simulink library "HANcoder_STM32_Target2018b"  (R2018b)
settings: Solver=ode45  StartTime=0.0  StopTime=10.0  RelTol=1e-3  EnableMultiTasking=on
libraries: simulink x3
(part 4 of 7)

== system HANcoder_STM32_Target2018b/STM32-E407/UDP ==
  UDP Client Send : Subsystem  Tag=HANcoder_TARGET_STM32_E407  mask(UDP Client Send){ip1=192, ip2=168, ip3=178, ip4=35, port=2000, inputNumber=10, dataType=uint8, byteOrder=on, tsamp=-1}
      mask prompts: ip1 "IP address 1"; ip2 "IP address 2"; ip3 "IP address 3"; ip4 "IP address 4"; inputNumber "Input ports"; dataType "Input datatype"; byteOrder "Byte order: Checked = MSB first, unchecked = LSB first."; tsamp "Sample time"
      mask help:
      | Function
      | ========
      | Sends a data packet to the UDP server with the specified IP address on
      | the specified port.
      |
      | Parameters
      | ==========
      | IP address 1:   First quad of the UDP server's IP address.
      | IP address 2:   Second quad of the UDP server's IP address.
      | IP address 3:   Third quad of the UDP server's IP address.
      | IP address 4:   Fourth quad of the UDP server's IP address.
      | Port:           Port to send the data packet on.
      | Input ports:    The amount of input ports.
      | Input datatype: The datatype of the input ports.
      | Byte order:     Select MSB or LSB first.
      | Sample time:    -1 or divisible by base sample time [seconds].
      |
      | Input
      | =====
      | Port 1..32      UDP packet data.
      mask init:
      | sfcn_udp_client_send_mcb(ip1,ip2,ip3,ip4,port,inputNumber,dataType,byteOrder);
      settings: MoveFcn=drawLogos
      mask Help: web('sfcn_udp_client_send.html');
      mask TypeOptions inputNumber: 1 | 2 | 3 | 4 | 5 | 6 | 7 | 8 | 9 | 10 | 11 | 12 | 13 | 14 | 15 | 16 | 17 | 18 | 19 | 20 | 21 | 22 | 23 | 24 | 25 | 26 | 27 | 28 | 29 | 30 | 31 | 32
      mask TypeOptions dataType: int8 | uint8 | int16 | uint16 | int32 | uint32 | boolean
      mask Display: fprintf('UDP Client Send\n\nport: %d\nip: %d.%d.%d.%d', port, ip1, ip2, ip3, ip4);patch([125 131 131],[8 14 2],[1 0 0]);patch([133 133 139],[14 2 8],[0 0 0.35]);
  UDP Server Init : Subsystem  Tag=HANcoder_TARGET_STM32_E407  mask(UDP Server Init){port=2001}
      mask help:
      | Function
      | ========
      | Initializes the UDP server to listen for and receive data packets on the
      | specified port.
      |
      | Parameters
      | ==========
      | Port:           Port to listen on.
      mask init:
      | sfcn_udp_server_init_mcb(port);
      settings: MoveFcn=drawLogos
      mask Help: web('sfcn_udp_server_init.html');
      mask Display: fprintf('UDP Server Init\n\nport: %d', port);patch([128 134 134],[8 14 2],[1 0 0]);patch([136 136 142],[14 2 8],[0 0 0.35]);
  UDP Server New Data Available : Subsystem  Tag=HANcoder_TARGET_STM32_E407  mask(UDP Server New Data Available){tsamp=-1}
      mask prompts: tsamp "Sample time"
      mask help:
      | Function
      | ========
      | Checks if the UDP server has new data in its internal receive buffer. This
      | new data flag is set each time a data packet is received by the UDP server.
      | It is reset when the application reads data from the receive buffer.
      |
      | Parameters
      | ==========
      | Sample time:    -1 or divisible by base sample time [seconds].
      |
      | Outport
      | ==========
      | 1 if new data is available in the UDP server's receive buffer that hasn't
      | been read yet by the application, 0 otherwise.
      mask init:
      | sfcn_udp_server_new_mcb();
      settings: MoveFcn=drawLogos
      mask Help: web('sfcn_udp_server_new.html');
      mask Display: fprintf('UDP Server New\nData Available');patch([128 134 134],[8 14 2],[1 0 0]);patch([136 136 142],[14 2 8],[0 0 0.35]);
  UDP Server Receive : Subsystem  Tag=HANcoder_TARGET_STM32_E407  mask(UDP Server Receive){outputNumber=10, dataType=uint8, byteOrder=on, startIdx=1, tsamp=-1}
      mask prompts: outputNumber "Output ports"; dataType "Output datatype"; byteOrder "Byte order: Checked = MSB first, unchecked = LSB first."; startIdx "Start index"; tsamp "Sample time"
      mask help:
      | Function
      | ========
      | Reads data from the UDP server's internal receive buffer.
      |
      | Parameters
      | ==========
      | Output ports:    The amount of output ports.
      | Output datatype: The datatype of the output ports.
      | Byte order:      Select MSB or LSB first.
      | Start index:     Start index in the server's buffer to start reading from.
      | Sample time:     -1 or divisible by base sample time [seconds].
      |
      | Output
      | ======
      | Port 1..32       UDP received packet data.
      mask init:
      | sfcn_udp_server_receive_mcb(outputNumber, dataType, byteOrder, startIdx);
      settings: MoveFcn=drawLogos
      mask Help: web('sfcn_udp_server_receive.html');
      mask TypeOptions outputNumber: 1 | 2 | 3 | 4 | 5 | 6 | 7 | 8 | 9 | 10 | 11 | 12 | 13 | 14 | 15 | 16 | 17 | 18 | 19 | 20 | 21 | 22 | 23 | 24 | 25 | 26 | 27 | 28 | 29 | 30 | 31 | 32
      mask TypeOptions dataType: int8 | uint8 | int16 | uint16 | int32 | uint32 | boolean
      mask TypeOptions startIdx: 1 | 2 | 3 | 4 | 5 | 6 | 7 | 8 | 9 | 10 | 11 | 12 | 13 | 14 | 15 | 16 | 17 | 18 | 19 | 20 | 21 | 22 | 23 | 24 | 25 | 26 | 27 | 28 | 29 | 30 | 31 | 32
      mask Display: fprintf('UDP Server Receive');patch([130 136 136],[8 14 2],[1 0 0]);patch([138 138 144],[14 2 8],[0 0 0.35]);
  UDP Server Receive Size : Subsystem  Tag=HANcoder_TARGET_STM32_E407  mask(UDP Server Receive Size){tsamp=-1}
      mask prompts: tsamp "Sample time"
      mask help:
      | Function
      | ========
      | Reads the size in bytes of the last UDP packet that was received by the
      | UDP server and stored in its internal receive buffer.
      |
      | Parameters
      | ==========
      | Sample time:    -1 or divisible by base sample time [seconds].
      |
      | Outport
      | ==========
      | Number of bytes currently stored in the UDP server's receive buffer.
      mask init:
      | sfcn_udp_server_count_mcb();
      settings: MoveFcn=drawLogos
      mask Help: web('sfcn_udp_server_count.html');
      mask Display: fprintf('UDP Server Receive\n Size');patch([128 134 134],[8 14 2],[1 0 0]);patch([136 136 142],[14 2 8],[0 0 0.35]);

== system HANcoder_STM32_Target2018b/STM32-E407/UDS ==
  UDS Get Key : Subsystem  Tag=HANcoder_TARGET_STM32_E407  mask(UDS Get Key){tsamp=-1}
      mask prompts: tsamp "Sample time"
      mask help:
      | Function
      | ==========
      | Reads the 32-bit key value that was received from the UDS tester.
      |
      | Outport
      | =======
      |  - Key value that was received from the UDS tester.
      mask init:
      | sfcn_uds_get_key_mcb();
      settings: MoveFcn=drawLogos
      mask Help: web('sfcn_uds_get_key.html');
      mask Display: fprintf('UDS Get Key');patch([65 71 71],[8 14 2],[1 0 0]);patch([73 73 79],[14 2 8],[0 0 0.35]);
  UDS Get Seed : Subsystem  Tag=HANcoder_TARGET_STM32_E407  mask(UDS Get Seed){tsamp=-1}
      mask prompts: tsamp "Sample time"
      mask help:
      | Function
      | ==========
      | Reads the 32-bit seed value to be used in the seed/key unlock sequence.
      |
      | Outport
      | =======
      |  - Seed value to be used in the seed/key unlock sequence.
      mask init:
      | sfcn_uds_get_seed_mcb();
      settings: MoveFcn=drawLogos
      mask Help: web('sfcn_uds_get_seed.html');
      mask Display: fprintf('UDS Get Seed');patch([65 71 71],[8 14 2],[1 0 0]);patch([73 73 79],[14 2 8],[0 0 0.35]);
  UDS Get Seed Event : Subsystem  Tag=HANcoder_TARGET_STM32_E407  mask(UDS Get Seed Event){}
      mask help:
      | Function
      | ========
      | A 'UDS Get Seed Event' block is needed when the parameter 'UDS seed/key
      | required' is set to TRUE (checked) in the 'UDS Init' block.
      |
      | This block has a function call output that gets triggered during a seed/key
      | sequence, when the UDS module needs a seed. The connected subsystem should
      | contain a 'UDS Set Seed' block to give the seed back to the UDS module.
      |
      | Outport
      | =======
      | Event
      |   Allows connection of a function call subsystem.
      mask init:
      | sfcn_uds_get_seed_event_mcb();
      settings: MoveFcn=drawLogos
      mask Help: web('sfcn_uds_get_seed_event.html');
      mask Display: fprintf('UDS Get Seed Event');patch([95 101 101],[8 14 2],[1 0 0]);patch([103 103 109],[14 2 8],[0 0 0.35]);
  UDS Init : Subsystem  Tag=HANcoder_TARGET_STM32_E407  mask(UDS Init){canChannel=CAN 1, canTxId=hex2dec('7E8'), canRxId=hex2dec('7E0'), tpBlockSize=4, tpSTmin=40, tpRxBuffSize=64, udsTxBuffSize=64, udsUseSeedKey=off}
      mask prompts: canChannel "CAN channel"; canTxId "CAN transmit ID"; canRxId "CAN receive ID"; tpBlockSize "TP blocksize"; tpSTmin "TP STmin"; tpRxBuffSize "TP reception buffer size"; udsTxBuffSize "UDS transmit buffer size"; udsUseSeedKey "UDS seed/key required"
      mask help:
      | Function
      | ==========
      | Initializes the Unified Diagnostic Services (UDS) communication module.
      |
      | Parameters
      | ==========
      | CAN channel: The CAN channel to communicate on
      | CAN transmit ID: CAN identifier for ECU to Tester
      | CAN receive ID: CAN identifier for Tester to ECU
      | TP blocksize: Number of CF's to receive before sending a FC
      | TP STmin: Min separation time (ms) expected between CF's
      | TP reception buffer size: Size of the buffer for TP receptions
      | UDS transmit buffer size: Size of the buffer for UDS/TP transmissions
      | UDS seed/key required: Requires a seed/key unlock sequence
      mask init:
      | sfcn_uds_init_mcb(canChannel, canTxId, canRxId, tpBlockSize, tpSTmin, tpRxBuffSize, udsTxBuffSize, udsUseSeedKey);
      settings: MoveFcn=drawLogos
      mask Help: web('sfcn_uds_init.html');
      mask TypeOptions canChannel: CAN 1 | CAN 2
      mask TypeOptions tpBlockSize: 1 | 2 | 3 | 4 | 5 | 6 | 7 | 8 | 9 | 10 | 11 | 12 | 13 | 14 | 15 | 16 | 17 | 18 | 19 | 20 | 21 | 22 | 23 | 24 | 25 | 26 | 27 | 28 | 29 | 30 | 31 | 32 | 33 | 34 | 35 | 36 | 37 | 38 | 39 | 40 | 41 | 42 | 43 | 44 | 45 | 46 | 47 | 48 | 49 | 50 | 51 | 52 | 53 | 54 | 55 | 56 | 57 | 58 | 59 | 60 | 61 | 62 | 63 | 64 | 65 | 66 | 67 | 68 | 69 | 70 | 71 | 72 | 73 | 74 | 75 | 76 | 77 | 78 | 79 | 80 | 81 | 82 | 83 | 84 | 85 | 86 | 87 | 88 | 89 | 90 | 91 | 92 | 93 | 94 | 95 | 96 | 97 | 98 | 99 | 100 | 101 | 102 | 103 | 104 | 105 | 106 | 107 | 108 | 109 | 110 | 111 | 112 | 113 | 114 | 115 | 116 | 117 | 118 | 119 | 120 | 121 | 122 | 123 | 124 | 125 | 126 | 127 | 128 | 129 | 130 | 131 | 132 | 133 | 134 | 135 | 136 | 137 | 138 | 139 | 140 | 141 | 142 | 143 | 144 | 145 | 146 | 147 | 148 | 149 | 150 | 151 | 152 | 153 | 154 | 155 | 156 | 157 | 158 | 159 | 160 | 161 | 162 | 163 | 164 | 165 | 166 | 167 | 168 | 169 | 170 | 171 | 172 | 173 | 174 | 175 | 176 | 177 | 178 | 179 | 180 | 181 | 182 | 183 | 184 | 185 | 186 | 187 | 188 | 189 | 190 | 191 | 192 | 193 | 194 | 195 | 196 | 197 | 198 | 199 | 200 | 201 | 202 | 203 | 204 | 205 | 206 | 207 | 208 | 209 | 210 | 211 | 212 | 213 | 214 | 215 | 216 | 217 | 218 | 219 | 220 | 221 | 222 | 223 | 224 | 225 | 226 | 227 | 228 | 229 | 230 | 231 | 232 | 233 | 234 | 235 | 236 | 237 | 238 | 239 | 240 | 241 | 242 | 243 | 244 | 245 | 246 | 247 | 248 | 249 | 250 | 251 | 252 | 253 | 254 | 255
      mask TypeOptions tpSTmin: 1 | 2 | 3 | 4 | 5 | 6 | 7 | 8 | 9 | 10 | 11 | 12 | 13 | 14 | 15 | 16 | 17 | 18 | 19 | 20 | 21 | 22 | 23 | 24 | 25 | 26 | 27 | 28 | 29 | 30 | 31 | 32 | 33 | 34 | 35 | 36 | 37 | 38 | 39 | 40 | 41 | 42 | 43 | 44 | 45 | 46 | 47 | 48 | 49 | 50 | 51 | 52 | 53 | 54 | 55 | 56 | 57 | 58 | 59 | 60 | 61 | 62 | 63 | 64 | 65 | 66 | 67 | 68 | 69 | 70 | 71 | 72 | 73 | 74 | 75 | 76 | 77 | 78 | 79 | 80 | 81 | 82 | 83 | 84 | 85 | 86 | 87 | 88 | 89 | 90 | 91 | 92 | 93 | 94 | 95 | 96 | 97 | 98 | 99 | 100 | 101 | 102 | 103 | 104 | 105 | 106 | 107 | 108 | 109 | 110 | 111 | 112 | 113 | 114 | 115 | 116 | 117 | 118 | 119 | 120 | 121 | 122 | 123 | 124 | 125 | 126 | 127 | 128 | 129 | 130 | 131 | 132 | 133 | 134 | 135 | 136 | 137 | 138 | 139 | 140 | 141 | 142 | 143 | 144 | 145 | 146 | 147 | 148 | 149 | 150 | 151 | 152 | 153 | 154 | 155 | 156 | 157 | 158 | 159 | 160 | 161 | 162 | 163 | 164 | 165 | 166 | 167 | 168 | 169 | 170 | 171 | 172 | 173 | 174 | 175 | 176 | 177 | 178 | 179 | 180 | 181 | 182 | 183 | 184 | 185 | 186 | 187 | 188 | 189 | 190 | 191 | 192 | 193 | 194 | 195 | 196 | 197 | 198 | 199 | 200 | 201 | 202 | 203 | 204 | 205 | 206 | 207 | 208 | 209 | 210 | 211 | 212 | 213 | 214 | 215 | 216 | 217 | 218 | 219 | 220 | 221 | 222 | 223 | 224 | 225 | 226 | 227 | 228 | 229 | 230 | 231 | 232 | 233 | 234 | 235 | 236 | 237 | 238 | 239 | 240 | 241 | 242 | 243 | 244 | 245 | 246 | 247 | 248 | 249 | 250 | 251 | 252 | 253 | 254 | 255
      mask Display:
      | fprintf('UDS Init\n(CAN %x)', canChannel);
      | patch([65 71 71],[8 14 2],[1 0 0]);patch([73 73 79],[14 2 8],[0 0 0.35]);
  UDS Set Key Verfied : Subsystem  Tag=HANcoder_TARGET_STM32_E407  mask(UDS Set Key Verified){tsamp=-1}
      mask prompts: tsamp "Sample time"
      mask help:
      | Function
      | ========
      | Informs the UDS module whether or not the key received from the UDS tester
      | is valid.
      |
      | Inport
      | ======
      |  - Set to TRUE in case the key was valid, FALSE otherwise.
      mask init:
      | sfcn_uds_set_key_verified_mcb();
      settings: MoveFcn=drawLogos
      mask Help: web('sfcn_uds_set_key_verified.html');
      mask Display: fprintf('UDS Set Key\nVerified');patch([65 71 71],[8 14 2],[1 0 0]);patch([73 73 79],[14 2 8],[0 0 0.35]);
  UDS Set Seed : Subsystem  Tag=HANcoder_TARGET_STM32_E407  mask(UDS Set Seed){tsamp=-1}
      mask prompts: tsamp "Sample time"
      mask help:
      | Function
      | ==========
      | Sets the 32-bit seed value to be used in the seed/key unlock sequence.
      |
      | Inport
      | ======
      |  - Seed value to be used in the seed/key unlock sequence.
      mask init:
      | sfcn_uds_set_seed_mcb();
      settings: MoveFcn=drawLogos
      mask Help: web('sfcn_uds_set_seed.html');
      mask Display: fprintf('UDS Set Seed');patch([65 71 71],[8 14 2],[1 0 0]);patch([73 73 79],[14 2 8],[0 0 0.35]);
  UDS Verify Key Event : Subsystem  Tag=HANcoder_TARGET_STM32_E407  mask(UDS Verify Key Event){}
      mask help:
      | Function
      | ========
      | A 'UDS Verify Key Event' block is needed when the parameter 'UDS seed/key
      | required' is set to TRUE (checked) in the 'UDS Init' block.
      |
      | This block has a function call output that gets triggered during a seed/key
      | sequence, when the UDS module received a 32-bit key from the tester that
      | needs to be verified. The connected subsystem should contain a 'UDS Set Key
      | Verfied' block to inform the UDS module if the received key was correct.
      |
      | Outport
      | =======
      | Event
      |   Allows connection of a function call subsystem.
      mask init:
      | sfcn_uds_verify_key_event_mcb();
      settings: MoveFcn=drawLogos
      mask Help: web('sfcn_uds_verify_key_event.html');
      mask Display: fprintf('UDS Verify Key Event');patch([95 101 101],[8 14 2],[1 0 0]);patch([103 103 109],[14 2 8],[0 0 0.35]);

== system HANcoder_STM32_Target2018b/STM32-P405/Analog Inputs ==
  Analog Input : Subsystem  Tag=HANcoder_TARGET_STM32_P405  mask(Analog Input){pinID=Port A pin 1, tsamp=-1, filtered=off}
      mask prompts: pinID "Input pin"; tsamp "Sample time"; filtered "Use over sampling and filtering (causes high CPU load)"
      mask help:
      | Function
      | ========
      | Reads the analog/digital conversion results of an analog input pin.
      |
      | Parameters
      | ==========
      | Input pin:
      |   Selects the analog input to read
      |
      | Outport
      | ==========
      | uint16 12-bit conversion results (0-4095).
      mask init:
      | pinIDInfoStr = sfcn_analog_in_mcb(3, pinID,0);
      settings: MoveFcn=drawLogos
      mask Help: web('sfcn_analog_in.html');
      mask TypeOptions pinID: Port A pin 1 | Port B pin 0 | Port B pin 1 | Port C pin 0 | Port C pin 1 | Port C pin 2 | Port C pin 3 | Port C pin 4 | Port C pin 5
      mask Display: fprintf('Analog Input\n%s', pinIDInfoStr);patch([135 141 141],[8 14 2],[1 0 0]);patch([143 143 149],[14 2 8],[0 0 0.35]);

== system HANcoder_STM32_Target2018b/STM32-P405/CAN ==
  CAN : Subsystem
      settings: MoveFcn=drawLogos
      mask Display: fprintf('CAN');patch([85 91 91],[8 14 2],[1 0 0]);patch([93 93 99],[14 2 8],[0 0 0.35]);
  CANopenNode : Subsystem
      settings: MoveFcn=drawLogos
      mask Display: fprintf('CANopenNode');patch([85 91 91],[8 14 2],[1 0 0]);patch([93 93 99],[14 2 8],[0 0 0.35]);

== system HANcoder_STM32_Target2018b/STM32-P405/Digital Inputs ==
  Digital Input : Subsystem  Tag=HANcoder_TARGET_STM32_P405  mask(Digital Input){pinID=Port C pin 10 (5V Tolerant), config=Pulldown, tsamp=-1}
      mask prompts: pinID "Input pin"; config "Configuration"; tsamp "Sample time"
      mask help:
      | Function
      | ========
      | Reads the state of a digital input pin.
      |
      | Parameters
      | ==========
      | Input pin:
      |   Selects the digital input to read
      | Configuration:
      |   Determines if the input is floating or is connected to an internal
      |   pull-up or pull-down resistor.
      |
      | Outport
      | ==========
      | State of the pin. 0 means logical low and 1 logical high
      mask init:
      | pinIDInfoStr = sfcn_digital_in_mcb(3, pinID, config);
      settings: MoveFcn=drawLogos
      mask Help: web('sfcn_digital_in.html');
      mask TypeOptions pinID: Port A pin 1 (5V Tolerant) | Port A pin 8 (5V Tolerant) | Port B pin 0 (5V Tolerant) | Port B pin 1 (5V Tolerant) | Port B pin 2 (5V Tolerant) | Port B pin 5 (5V Tolerant) | Port B pin 8 (5V Tolerant) | Port B pin 9 (5V Tolerant) | Port B pin 10 (5V Tolerant) | Port B pin 11 (5V Tolerant) | Port B pin 12 (5V Tolerant) | Port B pin 13 (5V Tolerant) | Port B pin 14 (5V Tolerant) | Port B pin 15 (5V Tolerant) | Port C pin 0 (5V Tolerant) | Port C pin 1 (5V Tolerant) | Port C pin 2 (5V Tolerant) | Port C pin 3 (5V Tolerant) | Port C pin 4 (5V Tolerant) | Port C pin 5 (5V Tolerant) | Port C pin 6 (5V Tolerant) | Port C pin 7 (5V Tolerant) | Port C pin 8 (5V Tolerant) | Port C pin 9 (5V Tolerant) | Port C pin 10 (5V Tolerant) | Port C pin 11 (5V Tolerant) | Port C pin 12 (5V Tolerant) | Port C pin 13 (5V Tolerant) | Port D pin 2 (5V Tolerant) | Port A pin 0 - BUTTON (5V Tolerant)
      mask TypeOptions config: Floating | Pullup | Pulldown
      mask Display: fprintf('Digital Input\n%s', pinIDInfoStr);patch([135 141 141],[8 14 2],[1 0 0]);patch([143 143 149],[14 2 8],[0 0 0.35]);

== system HANcoder_STM32_Target2018b/STM32-P405/Digital Outputs ==
  Digital Output : Subsystem  Tag=HANcoder_TARGET_STM32_P405  mask(Digital Output){pinID=Port C pin 12 (LED), config=Push pull, tsamp=-1}
      mask prompts: pinID "Output pin"; config "Configuration"; tsamp "Sample time"
      mask help:
      | Function
      | ========
      | Controls the state of a digital output pin.
      |
      | Parameters
      | ==========
      | Output pin:
      |   Selects the digital output to control
      | Configuration:
      |   Open drain (output float when digital high) or push-pull (output connected
      |   to Vcc when digital high).
      |
      | Inport
      | ==========
      | State of the pin. 0 means logical low and 1 logical high
      mask init:
      | pinIDInfoStr = sfcn_digital_out_mcb(3, pinID, config);
      settings: CopyFcn=sfcn_digital_out_chk();  MoveFcn=drawLogos
      mask Help: web('sfcn_digital_out.html');
      mask TypeOptions pinID: Port A pin 1 | Port A pin 8 | Port B pin 0 | Port B pin 1 | Port B pin 2 | Port B pin 5 | Port B pin 8 | Port B pin 9 | Port B pin 10 | Port B pin 11 | Port B pin 12 | Port B pin 13 | Port B pin 14 | Port B pin 15 | Port C pin 0 | Port C pin 1 | Port C pin 2 | Port C pin 3 | Port C pin 4 | Port C pin 5 | Port C pin 6 | Port C pin 7 | Port C pin 8 | Port C pin 9 | Port C pin 10 | Port C pin 11 | Port C pin 12 (LED) | Port C pin 13 | Port D pin 2
      mask Callback pinID: sfcn_digital_out_chk();
      mask TypeOptions config: Open drain | Push pull
      mask Display: fprintf('Digital Output\n%s', pinIDInfoStr);patch([135 141 141],[8 14 2],[1 0 0]);patch([143 143 149],[14 2 8],[0 0 0.35]);

== system HANcoder_STM32_Target2018b/STM32-P405/Error Handling ==
  Clear errors : Subsystem  Tag=HANcoder_TARGET_STM32_P405  mask(Clear errors){eepromString=Active}
      mask prompts: eepromString "Active or Stored error"
      mask help:
      | [Function]
      | Clears the active(RAM) or stored(EEPROM) errors.
      |
      | [Triggerport]
      | Connect the port to a trigger source to execute the block only when necessary.
      mask init:
      | sfcn_controller_error_clearerrors_mcb(eepromString)
      settings: MoveFcn=drawLogos
      mask Help: web('sfcn_controller_error_clearerrors.html');
      mask TypeOptions eepromString: Active | Stored
      mask Display: fprintf('Clear %s Errors', eepromString);patch([80 86 86],[8 14 2],[1 0 0]);patch([88 88 94],[14 2 8],[0 0 0.35]);
  Delete error : Subsystem  Tag=HANcoder_TARGET_STM32_P405  mask(Delete error){useInPorts=off, errorID=hex2dec('8000'), para=10}
      mask prompts: useInPorts "Use inports"; errorID "Error code"; para "Error parameter"
      mask help:
      | [Function]
      | Delete an error defined by error code and parameter
      | from RAM.
      | Error ID and parameter can be specified in the mask or with inports.
      |
      | [Parameters]
      | Error code
      | Error parameter
      |
      | [Inputs]
      | 1 - Error code [uint16]
      | 2 - Error parameter [uint8]
      |
      | [Triggerport]
      | Connect the port to a trigger source to execute the block only when necessary.
      mask init:
      | sfcn_controller_error_deleteerror_mcb(useInPorts, errorID, para)
      settings: MoveFcn=drawLogos
      mask Help: web('sfcn_controller_error_deleteerror.html');
      mask Display: fprintf('Delete error');patch([80 86 86],[8 14 2],[1 0 0]);patch([88 88 94],[14 2 8],[0 0 0.35]);
  Read active error : Subsystem  Tag=HANcoder_TARGET_STM32_P405  mask(Read active error){tsamp=-1}
      mask prompts: tsamp "Sample time"
      mask help:
      | Function
      | ==========
      | Read an active error from RAM.
      |
      | Inport
      | ==========
      | Input is the number of the error in the error list, which can be 1..64. UINT8
      |
      | Outports
      | ==========
      | 1: UINT8 - total amount of errors.
      | 2: UINT16 - error code.
      | 3: UINT8  - error parameter.
      | 4: UINT8  - occurrence count.
      | 5: UINT32 - last occurrence time since startup [milliseconds].
      |
      | Note that the requested error was set and read only if occurrence count > 0.
      mask init:
      | sfcn_controller_error_readerror_mcb(0)
      settings: MoveFcn=drawLogos
      mask Help: web('sfcn_controller_error_readerror.html');
      mask Display: fprintf('Read active error');patch([80 86 86],[8 14 2],[1 0 0]);patch([88 88 94],[14 2 8],[0 0 0.35]);
  Read stored error : Subsystem  Tag=HANcoder_TARGET_STM32_P405  mask(Read stored error){tsamp=-1}
      mask prompts: tsamp "Sample time"
      mask help:
      | Function
      | ==========
      | Read a stored error from EEPROM.
      |
      | Inport
      | ==========
      | Input is the number of the error in the error list, which can be 1..64. UINT8
      |
      | Outports
      | ==========
      | 1: UINT8 - total amount of errors.
      | 2: UINT16 - error code.
      | 3: UINT8  - error parameter.
      | 4: UINT8  - occurrence count.
      | 5: UINT32 - last occurrence time since startup [milliseconds].
      |
      | Note that the requested error was set and read only if occurrence count > 0.
      mask init:
      | sfcn_controller_error_readerror_mcb(1)
      settings: MoveFcn=drawLogos
      mask Help: web('sfcn_controller_error_readerror.html');
      mask Display: fprintf('Read stored error');patch([80 86 86],[8 14 2],[1 0 0]);patch([88 88 94],[14 2 8],[0 0 0.35]);
  Search active error : Subsystem  Tag=HANcoder_TARGET_STM32_P405  mask(Search active error){tsamp=-1}
      mask prompts: tsamp "Sample time"
      mask help:
      | Function
      | ==========
      | Searches for the erorr with the specified error Code and Param in RAM.
      |
      | Inport
      | ==========
      | 1: UINT16 - Error Code
      | 2: UINT8   - Error Parameter
      |
      | Outports
      | ==========
      | 1: UINT8   - occurrence count.
      | 2: UINT32 - last occurrence time since startup [milliseconds]
      |
      | Note that when occurrence count equals zero, the error is not found.
      mask init:
      | sfcn_controller_error_searcherror_mcb(0)
      settings: MoveFcn=drawLogos
      mask Help: web('sfcn_controller_error_searcherror.html');
      mask Display: fprintf('Search active error');patch([80 86 86],[8 14 2],[1 0 0]);patch([88 88 94],[14 2 8],[0 0 0.35]);
  Search stored error : Subsystem  Tag=HANcoder_TARGET_STM32_P405  mask(Search stored error){tsamp=-1}
      mask prompts: tsamp "Sample time"
      mask help:
      | Function
      | ==========
      | Searches for the erorr with the specified error Code and Param in EEPROM.
      |
      | Inport
      | ==========
      | 1: UINT16 - Error Code
      | 2: UINT8   - Error Parameter
      |
      | Outports
      | ==========
      | 1: UINT8   - occurrence count.
      | 2: UINT32 - last occurrence time since startup [milliseconds]
      |
      | Note that when occurrence count equals zero, the error is not found.
      mask init:
      | sfcn_controller_error_searcherror_mcb(1)
      settings: MoveFcn=drawLogos
      mask Help: web('sfcn_controller_error_searcherror.html');
      mask Display: fprintf('Search stored error');patch([80 86 86],[8 14 2],[1 0 0]);patch([88 88 94],[14 2 8],[0 0 0.35]);
  "Store error " : Subsystem  Tag=HANcoder_TARGET_STM32_P405  mask(Store error){useInPorts=off, errorCode=hex2dec('8000'), parameter=10}
      mask prompts: useInPorts "Use inports"; errorCode "Error code"
      mask help:
      | [Function]
      | Store an error to RAM (and EEPROM if new) of the controller.
      | Error ID and parameter can be specified in the mask or with inports.
      |
      | [Parameters]
      | Error code
      | Error parameter
      |
      | [Inputs]
      | 1 - Error code [uint16]
      | 2 - Error parameter [uint8]
      |
      | [Triggerport]
      | Connect the port to a trigger source to execute the block only when necessary.
      mask init:
      | sfcn_controller_error_storeerror_in_mcb(useInPorts, errorCode, parameter, 1)
      settings: MoveFcn=drawLogos
      mask Help: web('sfcn_controller_error_storeerror.html');
      mask Display: fprintf('Store error');patch([80 86 86],[8 14 2],[1 0 0]);patch([88 88 94],[14 2 8],[0 0 0.35]);
  Total Errors : Subsystem  Tag=HANcoder_TARGET_STM32_P405  mask(Total active or stored errors){eepromString=Active, tsamp=-1}
      mask prompts: eepromString "Active or Stored error"; tsamp "Sample time"
      mask help:
      | [Function]
      | Returns the total amount of active or stored errors
      |
      | [Parameters]
      | Active or Stored error [-]
      | sampleTime: [s]
      |
      | [Outputs]
      | Port 1 :Total number of errors [uint8]
      | Port 2 :Highest occuring severity [uint8]
      mask init:
      | sfcn_controller_error_totalerrors_mcb(eepromString, tsamp);
      settings: MoveFcn=drawLogos
      mask Help: web('sfcn_controller_error_totalerrors.html');
      mask TypeOptions eepromString: Active | Stored
      mask Display: fprintf('Total %s Errors', eepromString);patch([80 86 86],[8 14 2],[1 0 0]);patch([88 88 94],[14 2 8],[0 0 0.35]);

== system HANcoder_STM32_Target2018b/STM32-P405/File Logger ==
  File Logger Close : Subsystem  Tag=HANcoder_TARGET_STM32_P405  mask(File Logger Close){}
      mask help:
      | Function
      | ========
      | With the File Logger module active, the data values of the configured signals
      | are sampled at a fixed time interval and written to the log-file on the SD-card.
      |
      | The log-file needs to be explicitly closed at the end of a logging session for the
      | log-file to actually appear on the SD-card.
      |
      | Ideally, this block is called during software shutdown for example when the ignition
      | signal goes low in automotive applications. An external trigger can also be used such
      | as a button press event or CAN message reception.
      |
      | Triggerport
      | ===========
      | Connect the port to a trigger source to execute the block only when necessary.
      mask init:
      | sfcn_filelogger_close_mcb();
      settings: MoveFcn=drawLogos
      mask Help: web('sfcn_filelogger_close.html')
      mask Display: fprintf('File Logger Close');patch([80 86 86],[8 14 2],[1 0 0]);patch([88 88 94],[14 2 8],[0 0 0.35]);
  File Logger Init : Subsystem  Tag=HANcoder_TARGET_STM32_P405  mask(File Logger Init){filename=file.txt, interval=100, fileLoggerMaxFileLength=30, autostart=off, dotseparator=off}
      mask prompts: interval "Logging interval (ms)"; fileLoggerMaxFileLength "Maximum log file size (in KB)"; autostart "Automatically start logging"; dotseparator "Use dot-character as decimal separator (comma otherwise)"
      mask help:
      | Function
      | ==========
      | Initializes the File Logger module to log on the SDcard.
      |
      | Parameters per channel
      | ======================
      | - Filename for the log-file (a number will be added at the end of
      |   the filename for each new logfile)
      | - Logging interval in milliseconds
      | - Maximum size of the log file, a new log file will be started each time
      |   the file size is reached.
      | - Select if logging should automatically start after reset. If not then
      |   logging can be started using the trigger input.
      | - Select if a comma or dot should be used a the decimal point in numbers
      |
      | Note: Use the 'File Logger Close' block to save the data to the SDcard
      mask init:
      | sfcn_filelogger_init_mcb(filename, interval, dotseparator, autostart, fileLoggerMaxFileLength);
      settings: MoveFcn=drawLogos
      mask Help: web('sfcn_filelogger_init.html')
      mask Display: fprintf('File Logger Init');patch([95 101 101],[8 14 2],[1 0 0]);patch([103 103 109],[14 2 8],[0 0 0.35]);
  File Logger Signal : Subsystem  Tag=HANcoder_TARGET_STM32_P405  mask(File Logger Signal){signalName=enter name, dataType=uint8, defineColumns=off, columnNr=1}
      mask prompts: signalName "Signal Name"; dataType "Signal Data Type"; defineColumns "Define ALL column numbers manually"; columnNr "Column number starting at 1:"
      mask help:
      | Function
      | ==========
      | Configures the signal to be logged by the File Logger module.
      |
      | Parameters per channel
      | ======================
      | - Select the name for in the first line of the log file.
      | - Select the data type of the signal.
      | - Check if you want to give a column number to the signal or let Simulink
      |   automatically do it.
      | - Indicate the column in the logfile where this signal's data should be
      |   present (Note: you have to do all of your logged signals)
      settings: MoveFcn=drawLogos
      mask Help: web('sfcn_filelogger_signal.html')
      mask TypeOptions dataType: double | single | int8 | uint8 | int16 | uint16 | int32 | uint32
      mask Callback defineColumns:
      | if strcmp(get_param(gcb, 'defineColumns'),'on')
      | 	set_param(gcb, 'MaskVisibilities',{'on' 'on' 'on' 'on'});
      | else
      |     set_param(gcb, 'MaskVisibilities',{'on' 'on' 'on' 'off'});
      | end
      mask Display:
      | switch dataType
      |     case 1
      |         dataTypeStr = 'double';
      |     case 2
      |         dataTypeStr = 'single';
      |     case 3
      |         dataTypeStr = 'int8';
      |     case 4
      |         dataTypeStr = 'uint8';
      |     case 5
      |         dataTypeStr = 'int16';
      |     case 6
      |         dataTypeStr = 'uint16';
      |     case 7
      |         dataTypeStr = 'int32';
      |     case 8
      |         dataTypeStr = 'uint32';
      |     case 9
      |         dataTypeStr = 'boolean';
      | end
      | fprintf('File Logger Signal\n%s (%s)', signalName, dataTypeStr);patch([110 116 116],[8 14 2],[1 0 0]);patch([118 118 124],[14 2 8],[0 0 0.35]);

== system HANcoder_STM32_Target2018b/STM32-P405/Memory ==
  EEPROM : Subsystem
      settings: MoveFcn=drawLogos
      mask Display: fprintf('EEPROM');patch([85 91 91],[8 14 2],[1 0 0]);patch([93 93 99],[14 2 8],[0 0 0.35]);

== system HANcoder_STM32_Target2018b/STM32-P405/PWM Outputs ==
  PWM Duty Cycle : Subsystem  Tag=HANcoder_TARGET_STM32_P405  mask(Pulse Width Modulation Set Duty Cycle){pinID=Port A pin 9, tsamp=-1}
      mask prompts: pinID "Output pin"; tsamp "Sample time"
      mask help:
      | Function
      | ========
      | A 'PWM Duty Cycle' block allows the duty cycle of the generated PWM signal to
      | changed.
      | Note that this only works properly if a 'PWM Init' block is also present
      | for initializing the related PWM module.
      |
      | Parameters
      | ==========
      | PWM pin:
      |   Selects the PWM pin for which the duty cycle should be updated.
      |
      | Inport
      | ==========
      | uint16 10-bit unsigned value (0..1023) to represent the duty cycle (0..100%) for
      | each enabled channel.
      mask init:
      | pinIDInfoStr = sfcn_pwmout_setduty_mcb(3, pinID);
      settings: MoveFcn=drawLogos
      mask Help: web('sfcn_pwmout_setduty.html');
      mask TypeOptions pinID: Port A pin 8 | Port A pin 9 | Port A pin 10 | Port A pin 1 | Port C pin 6 | Port C pin 7 | Port C pin 8 | Port C pin 9 | Port B pin 6 | Port B pin 7 | Port B pin 8 | Port B pin 9
      mask Display: fprintf('PWM Set Duty Cycle\n%s', pinIDInfoStr);patch([135 141 141],[8 14 2],[1 0 0]);patch([143 143 149],[14 2 8],[0 0 0.35]);
  PWM Init : Subsystem  Tag=HANcoder_TARGET_STM32_P405  mask(Pulse Width Modulation Initialization){moduleID=TIM1: PA8 & PA9 & PA10 & n/a + N-channels PB13 & PB0 & PB1), frequency=10253, alignment=Edge aligned, enableIRQoutput=off, ch1On=off, ch1Pol=Active high, ch1Inv=off, ch2On=off, ch2Pol=Active high, ch2Inv=off, ch3On=off, ch3Pol=Active high, ch3Inv=off, ch4On=off, ch4Pol=Active high, ch4Inv=off}
      mask prompts: moduleID "PWM module"; frequency "Signal frequency [Hz]"; alignment "Signal alignment"; enableIRQoutput "Enable IRQ output"; ch1On "Generate PWM signal on channel 1"; ch1Pol "Select signal polarity"; ch1Inv "Enable inverted signal on additional output pin"; ch2On "Generate PWM signal on channel 2"; ch2Pol "Select signal polarity"; ch2Inv "Enable inverted signal on additional output pin"; ch3On "Generate PWM signal on channel 3"; ch3Pol "Select signal polarity"; ch3Inv "Enable inverted signal on additional output pin"; ch4On "Generate PWM signal on channel 4"; ch4Pol "Select signal polarity"; ch4Inv "Enable inverted signal on additional output pin"
      mask help:
      | Function
      | ========
      | A 'PWM Init' block configures one of the STM32 timer modules for PWM
      | functionality, allowing a PWM signal to be generated on up to 4 timer
      | channels and their associated output pins.
      |
      | Parameters
      | ==========
      | General - PWM module:
      |   Select the PWM module to use. The name in the combo box contains
      |   information about which pins on the target belong to this timer module.
      |   Also the first pin corresponds with the first channel and so on:
      |   TIMx: Ch1 & Ch2 & Ch3...
      |
      | General - Signal frequency:
      |   Determines the signal frequency in Hz. If you click 'Apply' after entering
      |   the desired frequency it will automatically be adjusted to the closest
      |   supported value.
      |
      | General - Signal Aligment:
      |   Determines the aligment of the signal. It can either be edge aligned or
      |   center aligned.
      |
      | General - Enable IRQ output
      |   Controls whether or not the IRQ output is available.
      |
      | Channel x - Generate PWM signal on channel x:
      |   Enable to configure the channel for PWM functionality so that the PWM signal
      |   is outputted on the channel's associated microcontroller pin.
      |
      | Channel x - Signal polarity:
      |   Selects the polarity of the signal.
      |
      | Channel x - Enable inverted signal on additional output pin:
      |   When enabled, a second PWM signal will be generated on an additional
      |   microcontroller pin where the signal is an exact inversion of the first signal.
      mask init:
      | moduleIDInfoStr = sfcn_pwmout_init_mcb(3, moduleID, frequency, alignment, enableIRQoutput, ch1On, ch2On, ch3On, ch4On, ch1Pol, ch2Pol, ch3Pol, ch4Pol, ch1Inv, ch2Inv, ch3Inv, ch4Inv);
      settings: CopyFcn=sfcn_pwmout_init_chk();  MoveFcn=drawLogos
      mask Help: web('sfcn_pwmout_init.html');
      mask TypeOptions moduleID: TIM1: PA8 & PA9 & PA10 & n/a + N-channels PB13 & PB0 & PB1) | TIM2:n/a & PA1 & n/a & n/a | TIM3: PC6 & PC7 & PC8 & PC9 | TIM4: PB6 & PB7 & PC8 & PB9
      mask Callback moduleID: sfcn_pwmout_init_chk();
      mask TypeOptions alignment: Edge aligned | Center aligned
      mask TypeOptions ch1Pol: Active high | Active low
      mask TypeOptions ch2Pol: Active high | Active low
      mask TypeOptions ch3Pol: Active high | Active low
      mask TypeOptions ch4Pol: Active high | Active low
      mask Display: fprintf('PWM Init\n%s', moduleIDInfoStr);patch([185 191 191],[8 14 2],[1 0 0]);patch([193 193 199],[14 2 8],[0 0 0.35]);

== system HANcoder_STM32_Target2018b/STM32-P405/SPI ==
  SPI master init : Subsystem  Tag=HANcoder_TARGET_STM32_P405  mask(SPI master init){channel=SPI1: UEXT 9 & 7 & 8 (PA5 & PA6 & PA7), speed=5250 kHz, polarity=Idle low, phase=Sample bit on 1st clock edge}
      mask prompts: speed "Communication speed"
      mask help:
      | Function
      | ==========
      | Initialized a SPI master channel.
      |
      | Parameters per channel
      | ======================
      | - Select channel
      | - Select communication speed
      | - Select clock signal polarity
      | - Select clock phase to sample a bit
      mask init:
      | spiChannelInfoStr = sfcn_spi_master_init_mcb(3, channel, speed, polarity, phase);
      settings: CopyFcn=sfcn_spi_master_init_chk();  MoveFcn=drawLogos
      mask Help: web('sfcn_spi_master_init.html')
      mask TypeOptions channel: SPI1: UEXT 9 & 7 & 8 (PA5 & PA6 & PA7) | SPI2: PB13 & PB14 & PB15
      mask Callback channel: sfcn_spi_master_init_chk();
      mask TypeOptions speed: 21000 kHz | 10500 kHz | 5250 kHz | 2625 kHz | 1312.5 kHz | 656.25 kHz | 328.125 kHz | 164.0625 kHz
      mask TypeOptions polarity: Idle low | Idle high
      mask TypeOptions phase: Sample bit on 1st clock edge | Sample bit on 2nd clock edge
      mask Display: fprintf('SPI master init\n%s', spiChannelInfoStr);patch([211 217 217],[8 14 2],[1 0 0]);patch([219 219 225],[14 2 8],[0 0 0.35]);
  SPI master transfer : Subsystem  Tag=HANcoder_TARGET_STM32_P405  Priority=1  mask(SPI master transfer){channel=SPI1: UEXT 9 & 7 & 8 (PA5 & PA6 & PA7), useSS=off, SSpin=Port A pin 1, SSenable=on, SSdisable=on, delayCycles=0, userPriority=1, tsamp=-1}
      mask prompts: useSS "Use slave select output"; SSpin "Slave select output pin"; SSenable "Enable slave select before transfer"; SSdisable "Disable slave select after transfer"; delayCycles "Delay cycles between slave select enable and transfer"; userPriority "Priority (use to set order of byte transfer, lowest number is executed first)"; tsamp "Sample time"
      mask help:
      | Function
      | ==========
      | Performs a byte transfer via SPI.
      |
      | Parameters per channel
      | ======================
      | - Select channel
      | - Select if a Slave Select output should be controlled
      |   * Select the Slave Select digital output pin
      |   * Select if the Slave Select should be made logic low before the transfer
      |   * Select if the Slave Select should be made logic high after the transfer
      |   * Enter the number of CPU cycles to delay between Slave Select enable and the transfer
      |
      | Inputs
      | ======
      | The byte value to send to the slave.
      |
      | Outputs
      | =======
      | The byte value received from the slave.
      mask init:
      | spiChannelInfoStr = sfcn_spi_master_transfer_mcb(3, channel, useSS, SSpin, SSenable, SSdisable, delayCycles);
      settings: MoveFcn=drawLogos
      mask Help: web('sfcn_spi_master_transfer.html')
      mask TypeOptions channel: SPI1: UEXT 9 & 7 & 8 (PA5 & PA6 & PA7) | SPI2: PB13 & PB14 & PB15
      mask Callback useSS:
      | % Get the mask parameter
      | useSS = get_param(gcb,'useSS');
      | 
      | if strcmp(useSS,'on')
      |     set_param(gcb,'MaskVisibilities',{'on','on','on','on','on','on','on','on'});
      | else
      |     set_param(gcb,'MaskVisibilities',{'on','on','off','off','off','off','on','on'});
      | end
      mask TypeOptions SSpin: Port A pin 1 | Port A pin 8 | Port B pin 0 | Port B pin 1 | Port B pin 2 | Port B pin 5 | Port B pin 8 | Port B pin 9 | Port B pin 10 | Port B pin 11 | Port B pin 12 | Port B pin 13 | Port B pin 14 | Port B pin 15 | Port C pin 0 | Port C pin 1 | Port C pin 2 | Port C pin 3 | Port C pin 4 | Port C pin 5 | Port C pin 6 | Port C pin 7 | Port C pin 8 | Port C pin 9 | Port C pin 10 | Port C pin 11 | Port C pin 12 (LED) | Port C pin 13 | Port D pin 2
      mask Callback userPriority:
      | userPriority = get_param(gcb, 'userPriority');
      | set_param(gcb,'Priority',userPriority);
      mask Display: fprintf('SPI master transfer\n%s', spiChannelInfoStr);patch([210 216 216],[8 14 2],[1 0 0]);patch([218 218 224],[14 2 8],[0 0 0.35]);

== system HANcoder_STM32_Target2018b/STM32-P405/System Config ==
  Base Sample Time config : Subsystem  Tag=HANcoder_TARGET_STM32_P405  Description=HANcoder Target STM32-P405 blockset version 1.1  mask(Base Sample Time config){baseSampleTime=10, extraStack=100}
      mask prompts: baseSampleTime "Define the base sample time [ms]"; extraStack "Additional task stack (bytes):"
      mask help:
      | Function
      | ==========
      | Sets the Base Sample Time in the model, and automatically sets the sample
      | time in the solver step time menu when the model is simulated or build.
      |
      | Parameters
      | ==========
      | Base Sample Time [milliseconds]
      | Default:    10[ms]
      | Min:        0.1[ms]
      |
      | Note: This is the only block where sample time is set in miliseconds,
      | all other blocks work with sample time in seconds
      |
      | It is possible to reserve extra stack space for the OS task that executes
      | the model on the embedded target (AppCtrlTask).
      mask init:
      | sfcn_base_sample_time_mcb(baseSampleTime*1000, extraStack, 3);
      | HANcoderStruct = get_param(gcb,'UserData');
      | BlocksetVersion = HANcoderStruct.BlocksetVersion;
      settings: MoveFcn=drawLogos
      mask Help: web('sfcn_base_sample_time.html')
      mask Display: fprintf('Blockset version %s\nBase Sample Time:\n %gms',BlocksetVersion,baseSampleTime);patch([91 97 97],[8 14 2],[1 0 0]);patch([99 99 105],[14 2 8],[0 0 0.35]);
  Build settings : Subsystem  Tag=HANcoder_TARGET_STM32_P405  mask(Build Settings){AutoASAP2add=on, AutoFlash=USB}
      mask prompts: AutoASAP2add "Add signals and parameters automatically"; AutoFlash "Automatic flash after build"
      mask help:
      | Function
      | ==========
      | Auto Add:
      | Here you can turn the automatic adding of Signals and Parameters on or off. If the option is on all the parameters and signals which are not defined in the workspace will be added. You will be prompted for the value.
      |
      | Auto Flash:
      | This option will automatically start MicroBoot with the selected interface.
      settings: MoveFcn=drawLogos
      mask Help: web('build_settings.html')
      mask TypeOptions AutoASAP2add: on | off
      mask TypeOptions AutoFlash: off | USB | CAN
      mask DialogControl ParameterTabVar0 Prompt: Auto Add
      mask DialogControl Control3 Prompt: With this option the undefined parameters and signals will automatically be added to the workspace for use with HANtune. You will be prompted for the parameter values.
      mask DialogControl ParameterTabVar01 Prompt: Auto Flash
      mask DialogControl Control2 Prompt: With this option you can choose to automatically start MicroBoot after the build is complete. MicroBoot will start flashing using the selected interface.
      mask Display: fprintf('Build settings\nAuto Add: %s\nAuto Flash: %s',AutoASAP2add, AutoFlash);patch([114 120 120],[8 14 2],[1 0 0]);patch([122 122 128],[14 2 8],[0 0 0.35]);
  CAN config : Subsystem  Tag=HANcoder_TARGET_STM32_P405  mask(CAN config){txBufSize=64, evBufSize=8, canBus1=on, baudRate1=500, rxMask1=hex2dec('00000000'), rxCode1=hex2dec('00000000'), rxMode1=Receive only 11-bit message identifiers, canBus2=off, baudRate2=500, rxMask2=hex2dec('00000000'), rxCode2=hex2dec('00000000'), rxMode2=Receive only 11-bit message identifiers}
      mask prompts: txBufSize "Transmit buffer size CAN bus (max 512)"; evBufSize "Event buffer size CAN bus (max 16)"; canBus1 "Use CAN bus 1"; baudRate1 "Baudrate CAN bus 1 (kbit/s)"; rxMask1 "Reception filter Mask CAN bus 1"; rxCode1 "Reception filter Code CAN bus 1"; rxMode1 "Reception filter Mode CAN bus 1"; canBus2 "Use CAN bus 2"; baudRate2 "Baudrate CAN bus 2 (kbit/s)"; rxMask2 "Reception filter Mask CAN bus 2"; rxCode2 "Reception filter Code CAN bus 2"; rxMode2 "Reception filter Mode CAN bus 2"
      mask help:
      | Function
      | ==========
      | Configures the settings for the STM32's CAN busses.
      |
      | Parameters per channel
      | ======================
      | - Activate channel
      | - Select baud rate (default 500[kbit/s])
      | - Select reception acceptance filter Code
      | - Select reception acceptance filter Mask
      | - Select reception acceptance filter Mode
      mask init:
      | sfcn_can_config_mcb(txBufSize, evBufSize, canBus1, baudRate1, rxMask1, rxCode1, rxMode1, canBus2, baudRate2, rxMask2, rxCode2, rxMode2);
      settings: MoveFcn=drawLogos
      mask Help: web('sfcn_can_config.html')
      mask TypeOptions baudRate1: 125 | 250 | 500 | 1000
      mask TypeOptions rxMode1: Receive only 11-bit message identifiers | Receive only 29-bit message identifiers | Received both 11- and 29-bit message identifiers
      mask TypeOptions baudRate2: 125 | 250 | 500 | 1000
      mask TypeOptions rxMode2: Receive only 11-bit message identifiers | Receive only 29-bit message identifiers | Received both 11- and 29-bit message identifiers
      mask DialogControl ParameterTabVar0 Prompt: Generic
      mask DialogControl ParameterTabVar01 Prompt: CAN 1
      mask DialogControl ParameterTabVar012 Prompt: CAN 2
      mask Display: fprintf('CAN1 : %x\nCAN2 : %x',canBus1, canBus2);patch([58 64 64],[8 14 2],[1 0 0]);patch([66 66 72],[14 2 8],[0 0 0.35]);
  Custom ID config : Subsystem  Tag=HANcoder_TARGET_STM32_P405  mask(Custom ID config){softID=softwareID, softNUM=1}
      mask prompts: softID "Software ID Name"; softNUM "Software Version Number"
      mask help:
      | Function:
      | =========
      | This block can be used to override the generated software ID as the current software version which is used for identification purposes.
      | It can also be used to add a version number behind the software ID.
      |
      | Details:
      | ========
      | If only a software version number is filled in, a software ID will be generated and the version number will be placed behind it.
      | Atleast one pf the fields has to be filled in.
      |
      | Parameters:
      | ===========
      | Software ID name:
      | Fill in the desired custom ID. Must fit in a UINT8
      | Software Version Number:
      | Fill in the desired version number. Must fit in a UINT8
      mask init:
      | sfcn_custom_version_config_mcb(softID, softNUM)
      settings: MoveFcn=drawLogos
      mask Help: web('sfcn_custom_ID_config.html')
      mask Display: fprintf('Custom software ID:\n "%s"\n Software version:\n "%s"', char(softID), char(softNUM));patch([112 118 118],[8 14 2],[1 0 0]);patch([120 120 126],[14 2 8],[0 0 0.35]);
  XCP on CAN config : Subsystem  Tag=HANcoder_TARGET_STM32_P405  mask(XCP on CAN config){canBus=CAN 1, croID=hex2dec('665'), dtoID=hex2dec('666')}
      mask prompts: canBus "CAN channel"; croID "CRO identifier"; dtoID "DTO identifier"
      mask help:
      | Function
      | ==========
      | Implements XCP communication into your application using the CAN network.
      |
      | Parameter
      | ==========
      | Specify the CAN channel to be used for XCP.
      | Specify the CAN CRO message identifier for XCP (master->slave).
      | Specify the CAN DTO message identifier for XCP (slave->master).
      |
      | Notes
      | ==========
      | Baudrates can be modified in the CAN config block.
      mask init:
      | sfcn_can_xcp_config_mcb(canBus, croID, dtoID)
      settings: MoveFcn=drawLogos
      mask Help: web('sfcn_can_xcp_config.html')
      mask TypeOptions canBus: CAN 1 | CAN 2
      mask Display: fprintf('XCP over CAN: %x',canBus);patch([69 75 75],[8 14 2],[1 0 0]);patch([77 77 83],[14 2 8],[0 0 0.35]);
  XCP on USB config : Subsystem  Tag=HANcoder_TARGET_STM32_P405  mask(XCP on USB config){}
      mask help:
      | Function
      | ==========
      | Implements XCP communication into your application using the USB Virtual COM-port.
      mask init:
      | sfcn_usb_xcp_config_mcb()
      settings: MoveFcn=drawLogos
      mask Help: web('sfcn_usb_xcp_config.html')
      mask Display: fprintf('XCP over USB');patch([69 75 75],[8 14 2],[1 0 0]);patch([77 77 83],[14 2 8],[0 0 0.35]);
